simulink model "Model_Full"  (R2015a)
settings: Solver=ode4  StartTime=0.0  StopTime=T_sim  FixedStep=0.01  RelTol=1e-3
values from neighbouring files (symbols this model uses):
  D1 = 1.333293908881934    (= 1.33329390888)    [NastawyPID.m]    (also in SzukanieNastaw.m = Nastawy(2); wskaznikJakosci.m = params(2); wskaznikJakosci2.m = params(2); wskaznikJakosciCzas.m = params(2))
  D2 = -0.189641732763578    (= -0.189641732764)    [NastawyPID.m]    (also in wskaznikJakosci.m = params(2); wskaznikJakosci2.m = params(4); wskaznikJakosciCzas.m = params(2))
  h0 = 5    [NastawyPID.m]    (also in wskaznikJakosci.m = 30; wskaznikJakosci2.m; wskaznikJakosciCzas.m = 30)
  I2 = 0    [NastawyPID.m]    (also in wskaznikJakosci.m; wskaznikJakosciCzas.m)
  P1 = 1.559211858494873    (= 1.55921185849)    [NastawyPID.m]    (also in SzukanieNastaw.m = Nastawy(1); wskaznikJakosci.m = params(1); wskaznikJakosci2.m = params(1); wskaznikJakosciCzas.m = params(1))
  P2 = 30.027479029282310    (= 30.0274790293)    [NastawyPID.m]    (also in wskaznikJakosci.m = params(1); wskaznikJakosci2.m = params(3); wskaznikJakosciCzas.m = params(1))
  zaworC2 = [-0.0843515690572 -0.078583483225 0.854642388664]    [parametryWielomianuC2Zaworu.mat]
undefined symbols (not defined in the file or in its folder): pompaP1, sigbuilder_block, zaworC1, zaworP1
libraries: simulink x3
settings Model: Creator=konra  LastModifiedBy=Kamil

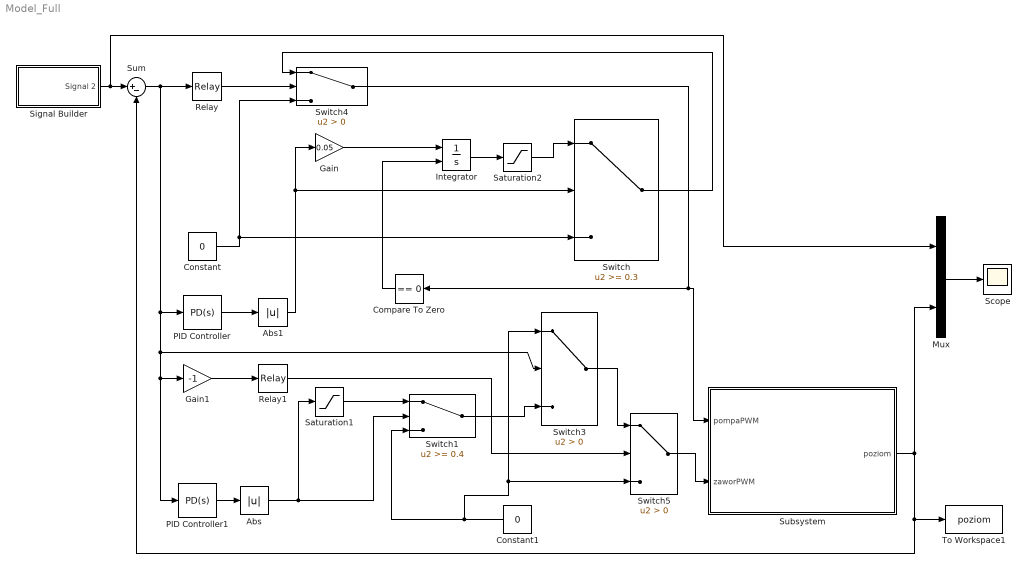
== system Model_Full ==
  Abs : Abs
  Abs1 : Abs
  Compare To Zero : simulink/Logic and Bit Operations/Compare To Zero  relop===  OutDataTypeStr=boolean
  Constant : Constant  Value=0
  Constant1 : Constant  Value=0
  Gain : Gain  Gain=0.05
  Gain1 : Gain  Gain=-1
  Integrator : Integrator  ExternalReset=level hold  InitialCondition=0.3
  Mux : Mux  Inputs=2
  PID Controller : simulink/Continuous/PID Controller  Controller=PD  TimeDomain=Continuous-time  SampleTime=-1  IntegratorMethod=Forward Euler  FilterMethod=Forward Euler  Form=Parallel  UseFilter=on  ControllerParametersSource=internal  P=P1  I=0.1  D=D1  N=100  InitialConditionSource=internal  InitialConditionForIntegrator=0  InitialConditionForFilter=0  ExternalReset=none  LimitOutput=on  UpperSaturationLimit=0.8  LowerSaturationLimit=0.3  LinearizeAsGain=on  AntiWindupMode=none  Kb=1  TrackingMode=off  Kt=1  PParamMin=[]  PParamMax=[]  IParamMin=[]  IParamMax=[]  DParamMin=[]  DParamMax=[]  NParamMin=[]  NParamMax=[]  KbParamMin=[]  KbParamMax=[]  KtParamMin=[]  KtParamMax=[]  POutMin=[]  POutMax=[]  IOutMin=[]  IOutMax=[]  DOutMin=[]  DOutMax=[]  NOutMin=[]  NOutMax=[]  KbOutMin=[]  KbOutMax=[]  KtOutMin=[]  KtOutMax=[]  IntegratorOutMin=[]  IntegratorOutMax=[]  FilterOutMin=[]  FilterOutMax=[]  SumOutMin=[]  SumOutMax=[]  SumI1OutMin=[]  SumI1OutMax=[]  SumI2OutMin=[]  SumI2OutMax=[]  SumI3OutMin=[]  SumI3OutMax=[]  SumDOutMin=[]  SumDOutMax=[]  SaturationOutMin=[]  SaturationOutMax=[]  IntegratorContinuousStateAttributes=''  IntegratorStateMustResolveToSignalObject=off  IntegratorRTWStateStorageClass=Auto  FilterContinuousStateAttributes=''  FilterStateMustResolveToSignalObject=off  FilterRTWStateStorageClass=Auto  DifferentiatorICPrevScaledInput=0  DifferentiatorOutMin=[]  DifferentiatorOutMax=[]
  PID Controller1 : simulink/Continuous/PID Controller  Controller=PD  TimeDomain=Continuous-time  SampleTime=-1  IntegratorMethod=Forward Euler  FilterMethod=Forward Euler  Form=Ideal  UseFilter=on  ControllerParametersSource=internal  P=P2  I=I2  D=D2  N=100  InitialConditionSource=internal  InitialConditionForIntegrator=0  InitialConditionForFilter=0  ExternalReset=none  LimitOutput=off  UpperSaturationLimit=inf  LowerSaturationLimit=-inf  LinearizeAsGain=on  AntiWindupMode=none  Kb=1  TrackingMode=off  Kt=1  PParamMin=[]  PParamMax=[]  IParamMin=[]  IParamMax=[]  DParamMin=[]  DParamMax=[]  NParamMin=[]  NParamMax=[]  KbParamMin=[]  KbParamMax=[]  KtParamMin=[]  KtParamMax=[]  POutMin=[]  POutMax=[]  IOutMin=[]  IOutMax=[]  DOutMin=[]  DOutMax=[]  NOutMin=[]  NOutMax=[]  KbOutMin=[]  KbOutMax=[]  KtOutMin=[]  KtOutMax=[]  IntegratorOutMin=[]  IntegratorOutMax=[]  FilterOutMin=[]  FilterOutMax=[]  SumOutMin=[]  SumOutMax=[]  SumI1OutMin=[]  SumI1OutMax=[]  SumI2OutMin=[]  SumI2OutMax=[]  SumI3OutMin=[]  SumI3OutMax=[]  SumDOutMin=[]  SumDOutMax=[]  SaturationOutMin=[]  SaturationOutMax=[]  IntegratorContinuousStateAttributes=''  IntegratorStateMustResolveToSignalObject=off  IntegratorRTWStateStorageClass=Auto  FilterContinuousStateAttributes=''  FilterStateMustResolveToSignalObject=off  FilterRTWStateStorageClass=Auto  DifferentiatorICPrevScaledInput=0  DifferentiatorOutMin=[]  DifferentiatorOutMax=[]
  Relay : Relay  OnSwitchValue=1  OffSwitchValue=-1
  Relay1 : Relay  OnSwitchValue=1  OffSwitchValue=-1
  Saturation1 : Saturate  UpperLimit=1  LowerLimit=0.4
  Saturation2 : Saturate  UpperLimit=0.8  LowerLimit=0.3
  Scope : Scope
      settings: YMin=5  YMax=30
  Signal Builder : Subsystem  Tag=STV Subsys  LoadFcn=sigbuilder_block('load');  StartFcn=sigbuilder_block('start');  StopFcn=sigbuilder_block('stop');  ClipboardFcn=sigbuilder_block('clipboard');  mask(Sigbuilder block){}
      mask help: Simulink:masks:SigbuilderBlock_MD
      mask init:
      | if ~strcmp(get_param(bdroot(gcbh),'SimulationStatus'),'stopped') tuvar = sigbuilder_block('maskInit'); end
      settings: CopyFcn=sigbuilder_block('copy');  DeleteFcn=sigbuilder_block('delete');  ModelCloseFcn=sigbuilder_block('modelClose');  PreSaveFcn=sigbuilder_block('preSave');  PauseFcn=sigbuilder_block('pause');  ContinueFcn=sigbuilder_block('continue');  NameChangeFcn=sigbuilder_block('namechange');  OpenFcn=sigbuilder_block('open',[437.6 199.2 550.4 400 ]);  CloseFcn=sigbuilder_block('close');
      mask Display: plot(0, 0, 100, 100,[2, 2, 32, 32, 2], [68, 8, 8, 68, 68],[32, 2], [38, 38], [32, 19, 2],[53, 60, 44], [32, 17, 17, 2],[16, 16, 31, 31]);txt = getActiveGroup(gcbh);text(2, 100, txt,'verticalAlignment', 'top');
  Subsystem : Subsystem
  Sum : Sum  Inputs=|+-
  Switch : Switch  Threshold=0.3
  Switch1 : Switch  Threshold=0.4
  Switch3 : Switch  Criteria=u2 > Threshold
  Switch4 : Switch  Criteria=u2 > Threshold
  Switch5 : Switch  Criteria=u2 > Threshold
  To Workspace1 : ToWorkspace  VariableName=poziom  SaveFormat=Structure With Time  SampleTime=-1
  wires:
  Subsystem/1(poziom) -> Mux/2, To Workspace1/1, Sum/2
  Constant/1 -> Switch4/3, Switch/3
  PID Controller/1 -> Abs1/1
  Abs1/1 -> Gain/1, Switch/2
  Mux/1 -> Scope/1
  Switch/1 -> Switch4/1
  Relay/1 -> Switch4/2
  Switch4/1 -> Subsystem/1(pompaPWM), Compare To Zero/1
  Saturation1/1 -> Switch1/1
  Switch1/1 -> Switch3/3
  Constant1/1 -> Switch3/1, Switch5/3, Switch1/3
  PID Controller1/1 -> Abs/1
  Switch3/1 -> Switch5/1
  Abs/1 -> Saturation1/1, Switch1/2
  Switch5/1 -> Subsystem/2(zaworPWM)
  Sum/1 -> Relay/1, PID Controller/1, PID Controller1/1, Gain1/1, Switch3/2
  Relay1/1 -> Switch5/2
  Gain1/1 -> Relay1/1
  Signal Builder/1(Signal 2) -> Sum/1, Mux/1
  Integrator/1 -> Saturation2/1
  Gain/1 -> Integrator/1
  Saturation2/1 -> Switch/1
  Compare To Zero/1 -> Integrator/2

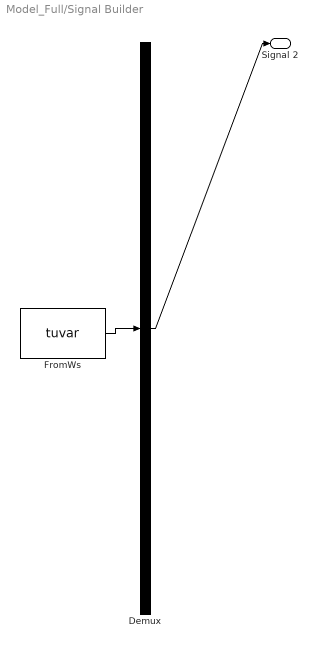
== system Model_Full/Signal Builder ==
  Demux : Demux  Tag=STV Demux  Outputs=1
  FromWs : FromWorkspace  Tag=STV FromWs  VariableName=tuvar  SampleTime=0
      SigBuilderData=|
      | common.afterFinalStr = 'Extrapolate'
      | common.sampleTime = 0
      | dataSet.timeRange = [0 300]
      | dataSet.name = 'Group 1'
      | sbobj.Groups.Name = 'Group 1'
      | sbobj.Groups.Signals.Name = 'Signal 2'
      | sbobj.Groups.Signals.XData = [0 80 80 200 200 300]
      | sbobj.Groups.Signals.YData = [30 30 20 20 25 25]
      | sbobj.Groups.TimeRange = [0 300]
  Signal 2 : Outport  Tag=STV Outport
  wires:
  FromWs/1 -> Demux/1
  Demux/1 -> Signal 2/1

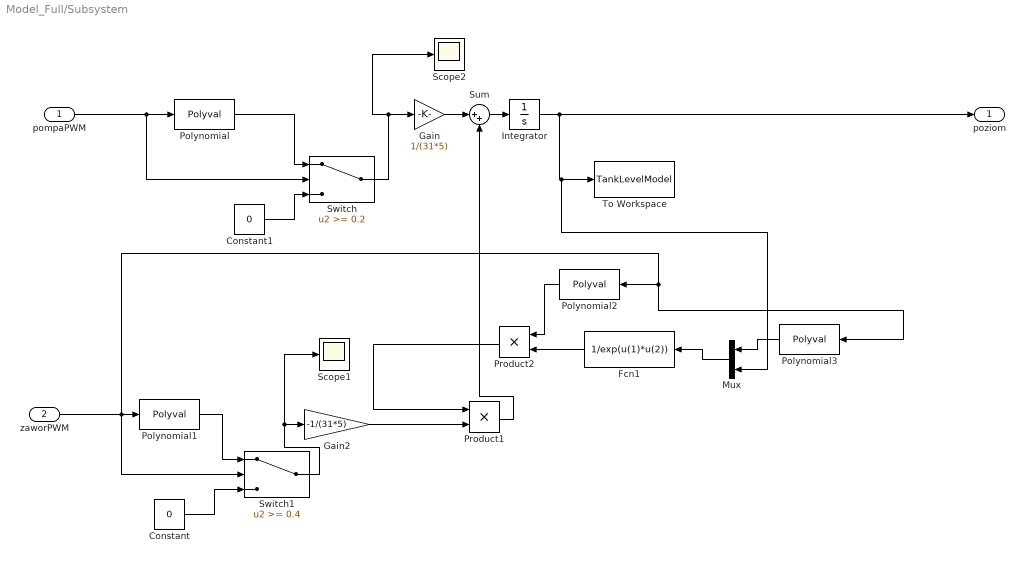
== system Model_Full/Subsystem ==
  pompaPWM : Inport
  zaworPWM : Inport  Port=2
  Constant : Constant  Value=0
  Constant1 : Constant  Value=0
  Fcn1 : Fcn  Expr=1/exp(u(1)*u(2))
  Gain : Gain  Gain=1/(31*5)
  Gain2 : Gain  Gain=-1/(31*5)
  Integrator : Integrator  InitialCondition=h0
  Mux : Mux  Inputs=2
  Polynomial : Polyval  Coefs=pompaP1
  Polynomial1 : Polyval  Coefs=zaworP1
  Polynomial2 : Polyval  Coefs=zaworC2
  Polynomial3 : Polyval  Coefs=zaworC1
  Product1 : Product
  Product2 : Product
  Scope1 : Scope
  Scope2 : Scope
      settings: SaveName=ScopeData2
  Sum : Sum  Inputs=|++
  Switch : Switch  Threshold=0.2
  Switch1 : Switch  Threshold=0.4
  To Workspace : ToWorkspace  VariableName=TankLevelModel  SaveFormat=Structure With Time  SampleTime=-1
  poziom : Outport
  wires:
  Switch1/1 -> Scope1/1, Gain2/1
  Polynomial1/1 -> Switch1/1
  Constant/1 -> Switch1/3
  Polynomial/1 -> Switch/1
  Constant1/1 -> Switch/3
  Switch/1 -> Scope2/1, Gain/1
  pompaPWM/1 -> Switch/2, Polynomial/1
  Gain2/1 -> Product1/2
  Product1/1 -> Sum/2
  Product2/1 -> Product1/1
  Integrator/1 -> poziom/1, Mux/2, To Workspace/1
  Fcn1/1 -> Product2/2
  zaworPWM/1 -> Switch1/2, Polynomial1/1, Polynomial3/1, Polynomial2/1
  Polynomial2/1 -> Product2/1
  Mux/1 -> Fcn1/1
  Polynomial3/1 -> Mux/1
  Gain/1 -> Sum/1
  Sum/1 -> Integrator/1
